simulink model "untitled"  (R2018a)
settings: Solver=VariableStepAuto  StartTime=0.0  StopTime=15  RelTol=1e-3
settings Model: Creator=HIBIKI  LastModifiedBy=HIBIKI

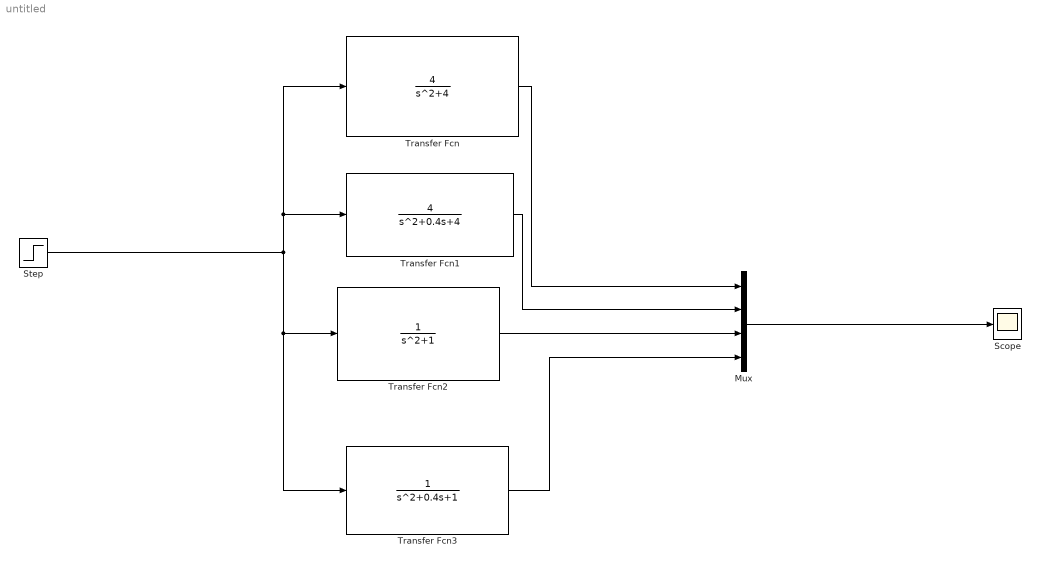
== system untitled ==
  Mux : Mux
  Scope : Scope
  Step : Step  Time=0  SampleTime=15
  Transfer Fcn : TransferFcn  Numerator=[4]  Denominator=[1 0 4]
  Transfer Fcn1 : TransferFcn  Numerator=[4]  Denominator=[1 0.4 4]
  Transfer Fcn2 : TransferFcn  Denominator=[1 0 1]
  Transfer Fcn3 : TransferFcn  Denominator=[1 0.4 1]
  wires:
  Transfer Fcn/1 -> Mux/1
  Transfer Fcn1/1 -> Mux/2
  Transfer Fcn2/1 -> Mux/3
  Transfer Fcn3/1 -> Mux/4
  Mux/1 -> Scope/1
  Step/1 -> Transfer Fcn3/1, Transfer Fcn2/1, Transfer Fcn/1, Transfer Fcn1/1
